simulink model "FAS_Kreuzungswarner_Simulation_V1"  (R2024b)
settings: Solver=FixedStepAuto  StartTime=0.0  StopTime=stoptime  FixedStep=sampletime  RelTol=1e-3
InitFcn:
  | if ~evalin('base', 'exist(''Auswertungsflag'', ''var'')') || evalin('base', 'Auswertungsflag.Value == 0')
  |     Parameterskript;
  |     run('StartGUI');  % explizit ausführen (nicht blockierend!)
  | end
values from neighbouring files (symbols this model uses):
  mEGO = str2double(massEGOInput.String)    [StartGUI.m]
  mFZG = str2double(massFZGInput.String)    [StartGUI.m]
  OeffnungswinkelA = str2double(angleInputA.String)    [StartGUI.m]
  OeffnungswinkelB = Simulink.Parameter    [Auswertung.m]    (also in StartGUI.m = str2double(angleInputB.String))
  P_EGO = str2double(powerEGOInput.String)    [StartGUI.m]
  P_FZG = str2double(powerFZGInput.String)    [StartGUI.m]
  ReichweiteA = str2double(rangeInputA.String)    [StartGUI.m]
  ReichweiteB = str2double(rangeInputB.String)    [StartGUI.m]
  SensorA = sensor1Dropdown.Value    [StartGUI.m]
  SensorB = sensor2Dropdown.Value    [StartGUI.m]
  startPositionEGO = str2double(posEGOInput.String)    [StartGUI.m]
  startPositionFzg = str2double(posFzgInput.String)    [StartGUI.m]
  v_EGO = str2double(velEGOInput.String)    [StartGUI.m]
  v_FZG = str2double(velFZGInput.String)    [StartGUI.m]
  Wetter = weatherDropdown.Value    [StartGUI.m]
  zweitesFzgSwitch = str2double(zweitesFzgInput.String)    [StartGUI.m]
undefined symbols (not defined in the file or in its folder): Airbagzeit, Ausloesezeit, b, dt, g, Haltezeit, l, munass, muschnee, mutrocken, rad_b, rad_l, reifen_dx, reifen_dy, SensorSwitch, startPositionFzg2, xFZG, yEGO
(part 2 of 3)

== matlab function FAS_Kreuzungswarner_Simulation_V1/FAF/MATLAB Function ==
  data: time input; Abstand input; GeschwindigkeitEGO input; Kollision input; Bremssignal input; Warnung input; defaultDistance parameter
%% Funktion zur Berechnung und Speicherung der für die Auswertung relevanten Parameter

% In dieser Funktion werden die für die Auswertung relevanten Parameter
% berechnet und danach im Workspace gespeichert sodass sie mit dem
% Auswertungsskript entsprechend gespeichert und dargestellt werden können

function Auswertung(time, Abstand, GeschwindigkeitEGO, Kollision, Bremssignal, Warnung, defaultDistance)
    
    persistent Kollisionszeitpunkt_gespeichert Erkennungszeitpunkt_gespeichert ReaktionszeitpunktWarnung_gespeichert ReaktionszeitpunktBremsung_gespeichert PufferzeitWarnung PufferzeitBremsung ...
                TimeToCollision Kollisionsgeschwindigkeit Kollisionszeitpunkt Erkennungszeitpunkt ReaktionszeitpunktWarnung ReaktionszeitpunktBremsung PufferAbstand

    % Variablen zur Berechnung der Zeitpunkte 
    if isempty(Kollisionszeitpunkt_gespeichert)
        Kollisionszeitpunkt_gespeichert = 0;
        Erkennungszeitpunkt_gespeichert = 0;
        ReaktionszeitpunktWarnung_gespeichert = 0;
        ReaktionszeitpunktBremsung_gespeichert = 0;
        Kollisionszeitpunkt = NaN;
        Erkennungszeitpunkt = NaN;
        ReaktionszeitpunktWarnung = NaN;
        ReaktionszeitpunktBremsung = NaN;
        PufferzeitWarnung = NaN;
        PufferzeitBremsung = NaN;
        TimeToCollision = NaN;
        Kollisionsgeschwindigkeit = NaN;
    end
    
    % Prüfung ob die Parameter einen Inhalt haben
    if isempty(PufferAbstand)
        PufferAbstand = defaultDistance;
    end

    if isempty(Kollisionszeitpunkt_gespeichert)
        Kollisionszeitpunkt_gespeichert = 0;
    end

    if isempty(Erkennungszeitpunkt_gespeichert)
        Erkennungszeitpunkt_gespeichert = 0;
    end

    if isempty(ReaktionszeitpunktWarnung_gespeichert)
        ReaktionszeitpunktWarnung_gespeichert = 0;
    end

    if isempty(ReaktionszeitpunktBremsung_gespeichert)
        ReaktionszeitpunktWarnung_gespeichert = 0;
    end
    
    % Wenn Kollision erkannt, Zeitpunkt nur einmal speichern
    if (Kollision > 0) && (Kollisionszeitpunkt_gespeichert == 0)
        Kollisionsgeschwindigkeit = GeschwindigkeitEGO * 3.6;
        Kollisionszeitpunkt = time;
        Kollisionszeitpunkt_gespeichert = 1;
    end

    % Erkennungszeitpunkt berechnen
    if (Abstand < defaultDistance) && (Erkennungszeitpunkt_gespeichert == 0)
        Erkennungszeitpunkt = time;
        Erkennungszeitpunkt_gespeichert = 1;
    end
    
    % Reaktionszeitpunkt für die Warnung berechnen
    if (Warnung > 0) && (ReaktionszeitpunktWarnung_gespeichert == 0)
        ReaktionszeitpunktWarnung = time;
        ReaktionszeitpunktWarnung_gespeichert = 1;
    end
    
    % Reaktionszeitpunkt für die Bremsung berechnen
    if (Bremssignal > 0) && (ReaktionszeitpunktBremsung_gespeichert == 0)
        ReaktionszeitpunktBremsung = time;
        ReaktionszeitpunktBremsung_gespeichert = 1;
    end    
    
    % Nur berechnen, wenn beide Zeitpunkte vorhanden sind
    if ~isnan(ReaktionszeitpunktWarnung) && ~isnan(Erkennungszeitpunkt)
        PufferzeitWarnung = ReaktionszeitpunktWarnung - Erkennungszeitpunkt;
    end

    if ~isnan(ReaktionszeitpunktBremsung) && ~isnan(Erkennungszeitpunkt)
        PufferzeitBremsung = ReaktionszeitpunktBremsung - Erkennungszeitpunkt;
    end
    
    if ~isnan(Kollisionszeitpunkt) && ~isnan(Erkennungszeitpunkt)
        TimeToCollision = Kollisionszeitpunkt - Erkennungszeitpunkt;
    end
    
    % Werte in Workspace schreiben (nur wenn diese gesetzt sind)
    if Kollisionszeitpunkt_gespeichert == 1
        assignin('base','Kollisionszeitpunkt',Kollisionszeitpunkt);
        assignin('base','Kollisionsgeschwindigkeit',Kollisionsgeschwindigkeit);
        Kollisionszeitpunkt_gespeichert = 2;
    end

    if Erkennungszeitpunkt_gespeichert == 1
        assignin('base','Erkennungszeitpunkt',Erkennungszeitpunkt);
        Erkennungszeitpunkt_gespeichert = 2;
    end

    if ReaktionszeitpunktWarnung_gespeichert == 1
        assignin('base','ReaktionszeitpunktWarnung',ReaktionszeitpunktWarnung);
        ReaktionszeitpunktWarnung_gespeichert = 2;
    end

    if ReaktionszeitpunktBremsung_gespeichert == 1
        assignin('base','ReaktionszeitpunktBremsung',ReaktionszeitpunktBremsung);
        ReaktionszeitpunktBremsung_gespeichert = 2;
    end

    if ~isnan(PufferzeitWarnung)
        assignin('base','PufferzeitWarnung',PufferzeitWarnung);
    end

    if ~isnan(PufferzeitBremsung)
        assignin('base','PufferzeitBremsung',PufferzeitBremsung);
    end
    
    % Werden auch bei NaN in den Workspace geschrieben da es Szenarien ohne
    % Crash gibt
    assignin('base','TimeToCollision',TimeToCollision);
    assignin('base','Kollisionszeitpunkt',Kollisionszeitpunkt);
    assignin('base','Kollisionsgeschwindigkeit',Kollisionsgeschwindigkeit);
    
    % PufferAbstand berechnen 
    if (PufferAbstand > Abstand)
        PufferAbstand = Abstand;
        assignin('base','PufferAbstand',PufferAbstand);
    end

== matlab function FAS_Kreuzungswarner_Simulation_V1/Sensor B/Radar/God Sensor mit Sichtfeld 1 ==
  data: xEGO input; yFzg input; distance output; collision output; yEGO parameter; xFZG parameter; b parameter; l parameter; OeffnungswinkelB parameter; ReichweiteB parameter
function [distance, collision] = abstand(xEGO, yFzg, yEGO, xFZG, b, l, OeffnungswinkelB, ReichweiteB)
    % Berechnung des Abstands zwischen EGO und Fzg, wenn Fzg sich im
    % Sichtfeld des EGO befindet

    % Initialisierung
    collision = 0;
    distance = 500;

    % Fahrzeugbegrenzungen berechnen
    x_min_Fzg = xFZG - b / 2;
    x_max_Fzg = xFZG + b / 2;
    y_min_Fzg = yFzg - l / 2;
    y_max_Fzg = yFzg + l / 2;
    x_min_EGO = xEGO - l / 2;
    x_max_EGO = xEGO + l / 2;
    y_min_EGO = yEGO - b / 2;
    y_max_EGO = yEGO + b / 2;

    % Kollisionsprüfung: Überlappung der Rechtecke?
    if (x_max_EGO >= x_min_Fzg && x_min_EGO <= x_max_Fzg) && ...
       (y_max_EGO >= y_min_Fzg && y_min_EGO <= y_max_Fzg)
        distance = 0;  
        collision = 10; % Kollision erkannt
        return
    end


    % Ecken + Kantenpunkte + Mittlepunkt des Fzg zur Sichtfeldprüfung
    testPoints = [
        linspace(x_min_Fzg, x_max_Fzg, 20)', repmat(y_min_Fzg, 20, 1); % Unterseite des Fzg
        linspace(x_min_Fzg, x_max_Fzg, 20)', repmat(y_max_Fzg, 20, 1); % Oberseite des Fzg
        repmat(x_min_Fzg, 18, 1), linspace(y_min_Fzg, y_max_Fzg, 18)'; % Linke Seite des Fzg
        repmat(x_max_Fzg, 18, 1), linspace(y_min_Fzg, y_max_Fzg, 18)'  % Rechte Seite des Fzg
        xFZG, yFzg % Mittelpunkt des Fzg
    ];

    % Sichtfeldprüfung: Mindestens ein Punkt im Sektor?
    isInside = false;
    for i = 1:size(testPoints,1)
        if isPointInSector(xEGO, yEGO, l, testPoints(i,1), testPoints(i,2), OeffnungswinkelB, ReichweiteB)
            isInside = true;
            break;
        end
    end

    if isInside
        if (collision ~= 10)
            % Messpunkte
            % EGO-Fahrzeug (horizontal ausgerichtet)
            top_EGO    = [linspace(x_min_EGO, x_max_EGO, 8)', repmat(y_max_EGO, 8, 1)];
            right_EGO  = [repmat(x_max_EGO, 8, 1), linspace(y_max_EGO, y_min_EGO, 8)'];
            bottom_EGO = [linspace(x_max_EGO, x_min_EGO, 8)', repmat(y_min_EGO, 8, 1)];
            left_EGO   = [repmat(x_min_EGO, 8, 1), linspace(y_min_EGO, y_max_EGO, 8)'];
            corners_EGO = [top_EGO; right_EGO; bottom_EGO; left_EGO];
    
            % Anderes Fahrzeug (vertikal ausgerichtet)
            top_Fzg    = [linspace(x_min_Fzg, x_max_Fzg, 8)', repmat(y_max_Fzg, 8, 1)];
            right_Fzg  = [repmat(x_max_Fzg, 8, 1), linspace(y_max_Fzg, y_min_Fzg, 8)'];
            bottom_Fzg = [linspace(x_max_Fzg, x_min_Fzg, 8)', repmat(y_min_Fzg, 8, 1)];
            left_Fzg   = [repmat(x_min_Fzg, 8, 1), linspace(y_min_Fzg, y_max_Fzg, 8)'];
            corners_Fzg = [top_Fzg; right_Fzg; bottom_Fzg; left_Fzg];
    
            % Abstand zwischen allen Punkten berechnen
            min_distance = inf;  
            for i = 1:32
                for j = 1:32
                    dx = corners_EGO(i,1) - corners_Fzg(j,1);
                    dy = corners_EGO(i,2) - corners_Fzg(j,2);
                    dist = sqrt(dx^2 + dy^2);
                    if dist < min_distance
                        min_distance = dist;
                    end
                end
            end
            distance = min_distance;
        end
    end
end

%% Sichtfeldprüfung für einen einzelnen Punkt
function isInside = isPointInSector(xEGO, yEGO, l, xP, yP, OeffnungswinkelB, ReichweiteB)
    % Prüft, ob der Punkt (xP, yP) im Sichtfeld des EGO liegt

    % Parameter
    OeffnungswinkelB = deg2rad(OeffnungswinkelB);
    alpha = -(OeffnungswinkelB/2);  % Startwinkel relativ zur x-Achse
    tol = max(1e-3, 1e-6 * ReichweiteB);

    % Mittelpunkt des Sektors
    xC = xEGO + l/2;
    yC = yEGO;

    % Richtungsvektor zum Punkt
    CP = [xP - xC, yP - yC];
    dist2 = CP(1)^2 + CP(2)^2;

    if dist2 > ReichweiteB^2 + tol
        isInside = false;
        return;
    end

    % Winkel vom Zentrum zum Punkt (in [-pi, pi])
    theta = atan2(CP(2), CP(1));  % atan2(y, x)

    % Endwinkel des Sichtfelds
    alphaEnd = alpha + OeffnungswinkelB;

    % Prüfung, ob Winkel theta im Sichtfeld liegt (inkl. Toleranz)
    isInside = (theta >= alpha - tol) && (theta <= alphaEnd + tol);
end

== matlab function FAS_Kreuzungswarner_Simulation_V1/Fahrdynamik/MATLAB Function ==
  data: VorgabeGeschwindigkeitEGO input; Anfahrgeschwindigkeit input; GeschwindigkeitEGO input; Geschwindigkeit_EGOneudelay input; Geschwindigkeit_EGOneu output
%% Berechnung der Geschwindigkeit des EGOs beim Anfahren

% Es wird die aktuelle Geschwindigkeit gespeichert solang sie niedriger ist
% als die Gschwindigkeit aus dem vorigen Simulationsschritt. Die minimale
% Geschwindigkeit wird gespeichert und mit der aktuellen
% Anfahrgeschwindigkeit verrechnet

function Geschwindigkeit_EGOneu = Geschwindigkeitsberechnung(VorgabeGeschwindigkeitEGO, Anfahrgeschwindigkeit, GeschwindigkeitEGO, Geschwindigkeit_EGOneudelay)

persistent Counter DummyGeschwindigkeit

% Prüfung ob Parameter schon einen Inhalt haben
if isempty(Counter)
    Counter = 0;
end

if isempty(DummyGeschwindigkeit)
    DummyGeschwindigkeit = 100000000;
end

% Prüfung ob die aktuelle Geschwindigkeit kleiner als die davor ist
if (DummyGeschwindigkeit > GeschwindigkeitEGO)
    DummyGeschwindigkeit = GeschwindigkeitEGO;
end

% Counter erhöhen, da der Integrator vor dem Berechnen nochmal auf 0
% gesetzt wird
if(Anfahrgeschwindigkeit == 0)
    Counter = Counter + 1;
end

% Verrechnen mit der Anfahrgeschwindigkeit beim Anfahren nach dem
% Bremsvorgang
if(Counter > 1 && VorgabeGeschwindigkeitEGO > Geschwindigkeit_EGOneudelay)
    Geschwindigkeit_EGOneu = Anfahrgeschwindigkeit + DummyGeschwindigkeit;
else
    Geschwindigkeit_EGOneu = GeschwindigkeitEGO;
end

== matlab function FAS_Kreuzungswarner_Simulation_V1/Sensor A/C2X/God Sensor mit Sichtfeld ==
  data: xEGO input; yFzg input; distance output; collision output; yEGO parameter; xFZG parameter; b parameter; l parameter; ReichweiteA parameter; relevanz input; OeffnungswinkelA parameter
function [distance, collision] = abstand(xEGO, yFzg, yEGO, xFZG, b, l, ReichweiteA, relevanz, OeffnungswinkelA)
    % Berechnung des Abstands zwischen EGO und Fzg, wenn Fzg sich im
    % Sichtfeld des EGO befindet
    % Initialisierung
    collision = 0;
    distance = 500;
    
    if relevanz == 1
        % Fahrzeugbegrenzungen berechnen
        x_min_Fzg = xFZG - b / 2;
        x_max_Fzg = xFZG + b / 2;
        y_min_Fzg = yFzg - l / 2;
        y_max_Fzg = yFzg + l / 2;
        x_min_EGO = xEGO - l / 2;
        x_max_EGO = xEGO + l / 2;
        y_min_EGO = yEGO - b / 2;
        y_max_EGO = yEGO + b / 2;

        % Kollisionsprüfung: Überlappung der Rechtecke?
        if (x_max_EGO >= x_min_Fzg && x_min_EGO <= x_max_Fzg) && ...
           (y_max_EGO >= y_min_Fzg && y_min_EGO <= y_max_Fzg)
            distance = 0;  
            collision = 10; % Kollision erkannt
            return
        end
    
        % Ecken + Kantenpunkte + Mittlepunkt des Fzg zur Sichtfeldprüfung
        testPoints = [
            linspace(x_min_Fzg, x_max_Fzg, 20)', repmat(y_min_Fzg, 20, 1); % Unterseite des Fzg
            linspace(x_min_Fzg, x_max_Fzg, 20)', repmat(y_max_Fzg, 20, 1); % Oberseite des Fzg
            repmat(x_min_Fzg, 18, 1), linspace(y_min_Fzg, y_max_Fzg, 18)'; % Linke Seite des Fzg
            repmat(x_max_Fzg, 18, 1), linspace(y_min_Fzg, y_max_Fzg, 18)'  % Rechte Seite des Fzg
            xFZG, yFzg % Mittelpunkt des Fzg
        ];
    
        % Sichtfeldprüfung: Mindestens ein Punkt im Sektor?
        isInside = false;
        for i = 1:size(testPoints,1)
            if isPointInSector(xEGO, yEGO, l, testPoints(i,1), testPoints(i,2), OeffnungswinkelA, ReichweiteA)
                isInside = true;
                break;
            end
        end
    
        if isInside
            if(collision ~= 10)
                % Messpunkte
                % EGO-Fahrzeug (horizontal ausgerichtet)
                top_EGO    = [linspace(x_min_EGO, x_max_EGO, 8)', repmat(y_max_EGO, 8, 1)];
                right_EGO  = [repmat(x_max_EGO, 8, 1), linspace(y_max_EGO, y_min_EGO, 8)'];
                bottom_EGO = [linspace(x_max_EGO, x_min_EGO, 8)', repmat(y_min_EGO, 8, 1)];
                left_EGO   = [repmat(x_min_EGO, 8, 1), linspace(y_min_EGO, y_max_EGO, 8)'];
                corners_EGO = [top_EGO; right_EGO; bottom_EGO; left_EGO];
        
                % Anderes Fahrzeug (vertikal ausgerichtet)
                top_Fzg    = [linspace(x_min_Fzg, x_max_Fzg, 8)', repmat(y_max_Fzg, 8, 1)];
                right_Fzg  = [repmat(x_max_Fzg, 8, 1), linspace(y_max_Fzg, y_min_Fzg, 8)'];
                bottom_Fzg = [linspace(x_max_Fzg, x_min_Fzg, 8)', repmat(y_min_Fzg, 8, 1)];
                left_Fzg   = [repmat(x_min_Fzg, 8, 1), linspace(y_min_Fzg, y_max_Fzg, 8)'];
                corners_Fzg = [top_Fzg; right_Fzg; bottom_Fzg; left_Fzg];
        
                % Abstand zwischen allen Punkten berechnen
                min_distance = inf;  
                for i = 1:32
                    for j = 1:32
                        dx = corners_EGO(i,1) - corners_Fzg(j,1);
                        dy = corners_EGO(i,2) - corners_Fzg(j,2);
                        dist = sqrt(dx^2 + dy^2);
                        if dist < min_distance
                            min_distance = dist;
                        end
                    end
                end
                distance = min_distance;
            end
        end
    end
end

%% Sichtfeldprüfung für einen einzelnen Punkt
function isInside = isPointInSector(xEGO, yEGO, l, xP, yP, OeffnungswinkelA, ReichweiteA)
    % Prüft, ob der Punkt (xP, yP) im Sichtfeld des EGO liegt

    % Parameter
    OeffnungswinkelA = deg2rad(OeffnungswinkelA);
    alpha = -(OeffnungswinkelA/2);  % Startwinkel relativ zur x-Achse
    tol = max(1e-3, 1e-6 * ReichweiteA);

    % Mittelpunkt des Sektors
    xC = xEGO + l/2;
    yC = yEGO;

    % Richtungsvektor zum Punkt
    CP = [xP - xC, yP - yC];
    dist2 = CP(1)^2 + CP(2)^2;

    if dist2 > ReichweiteA^2 + tol
        isInside = false;
        return;
    end

    % Winkel vom Zentrum zum Punkt (in [-pi, pi])
    theta = atan2(CP(2), CP(1));  % atan2(y, x)

    % Endwinkel des Sichtfelds
    alphaEnd = alpha + OeffnungswinkelA;

    % Prüfung, ob Winkel theta im Sichtfeld liegt (inkl. Toleranz)
    isInside = (theta >= alpha - tol) && (theta <= alphaEnd + tol);
end

== matlab function FAS_Kreuzungswarner_Simulation_V1/Sensor A/C2X/Relevanz Kontrolle/Bewegungs-Achse Fzg ==
  data: xFzg input; bewegung output; xFzg_prev input; yFzg input; yFzg_prev input
function bewegung = fcn(xFzg, xFzg_prev, yFzg, yFzg_prev)
% Prüfung ob Fzg eine Bewegung in X oder Y Richtung hat 
% X Bewegung: bewegung = 1
% Y Bewegung: bewegung = 2
% X&Y Bewegung: bewegung = 3
% Keine Bewegung: bewegung = 0

    if xFzg ~= xFzg_prev
        xBewegung = 1;
    else
        xBewegung = 0;
    end

    if yFzg  ~= yFzg_prev
        yBewegung = 2;
    else
        yBewegung = 0;
    end

    bewegung = xBewegung + yBewegung;

end

== matlab function FAS_Kreuzungswarner_Simulation_V1/Sensor A/C2X/Relevanz Kontrolle/Logik ==
  data: outY input; distance input; outX input; relevanz output; defaultDistance parameter
function relevanz = direction(outY, distance, outX, defaultDistance)
% Wenn der Sensor ein fzg erkennt (distance < defaultDistance) Wir wenn
% EGO und Fzg noch vor der Kreuzung sind eine Relevanz ausgegeben (1). Wenn
% nicht wird das Fzg als nicht Relevant gemarkt (-1)

    if distance < defaultDistance 
        if outX == 1 && outY == 1
            relevanz = 1;
        else
            relevanz = -1;
        end
    else
        relevanz = 0;
    end

end

== matlab function FAS_Kreuzungswarner_Simulation_V1/Sensor A/C2X/Relevanz Kontrolle/Relevanz Kreuzung x ==
  data: xPos input; out output; xPos_prev input; targetX input; b parameter
function out = direction(xPos, xPos_prev, targetX, b)
% Gibt 1 aus, wenn sich das Rechteck zubewegt oder innerhalb 4.25 ist
% Gibt -1 aus, wenn es sich entfernt und weiter als 4.25 ist
% Gibt 0 aus, wenn es genau auf dem Punkt ist

    % Berechne die Distanz des Rechtecks zum Zielpunkt targetY
    dist = abs(xPos - targetX);
    dist_prev = abs(xPos_prev - targetX);

    % Bewegungsrichtung des Rechtecks
    delta = dist - dist_prev;

    % Überprüfe die Bedingungen basierend auf der Bewegungsrichtung
    if dist <= b
        out = 1; % Rechteck bewegt sich auf den Punkt zu oder ist nah genug dran
    elseif delta < 0
        out = 1; % Rechteck bewegt sich auf den Punkt zu
    else
        out = -1; % Rechteck entfernt sich vom Punkt
    end
end

== matlab function FAS_Kreuzungswarner_Simulation_V1/Sensor A/C2X/Relevanz Kontrolle/Relevanz Kreuzung y ==
  data: yPos input; out output; yPos_prev input; targetY input; b parameter
function out = direction(yPos, yPos_prev, targetY, b)
% Gibt 1 aus, wenn sich das Rechteck zubewegt oder innerhalb 4.25 ist
% Gibt -1 aus, wenn es sich entfernt und weiter als 4.25 ist
% Gibt 0 aus, wenn es genau auf dem Punkt ist

    % Berechne die Distanz des Rechtecks zum Zielpunkt targetY
    dist = abs(yPos - targetY);
    dist_prev = abs(yPos_prev - targetY);

    % Bewegungsrichtung des Rechtecks
    delta = dist - dist_prev;

    % Überprüfe die Bedingungen basierend auf der Bewegungsrichtung
    if dist <= b
        out = 1; % Rechteck bewegt sich auf den Punkt zu oder ist nah genug dran
    elseif delta < 0
        out = 1; % Rechteck bewegt sich auf den Punkt zu
    else
        out = -1; % Rechteck entfernt sich vom Punkt
    end
end

== matlab function FAS_Kreuzungswarner_Simulation_V1/Sensor A/God Sensor/God Sensor ==
  data: xEGO input; yFzg input; distance output; collision output; yEGO parameter; xFZG parameter; b parameter; l parameter
function [distance, collision] = fcn(xEGO, yFzg, yEGO, xFZG, b, l)

    collision = 0;

    % Fahrzeugbegrenzungen berechnen
    x_min_EGO = xEGO - l / 2;
    x_max_EGO = xEGO + l / 2;
    y_min_EGO = yEGO - b / 2;
    y_max_EGO = yEGO + b / 2;

    x_min_Fzg = xFZG - b / 2;
    x_max_Fzg = xFZG + b / 2;
    y_min_Fzg = yFzg - l / 2;
    y_max_Fzg = yFzg + l / 2;

    % Kollisionsprüfung: Überlappen sich die Rechtecke?
    if (x_max_EGO >= x_min_Fzg && x_min_EGO <= x_max_Fzg) && ...
       (y_max_EGO >= y_min_Fzg && y_min_EGO <= y_max_Fzg)
        distance = 0;  
        collision = 10; % Kollision erkannt
        return
    else
        % Messpunkte
        % EGO-Fahrzeug (horizontal ausgerichtet)
        top_EGO    = [linspace(x_min_EGO, x_max_EGO, 8)', repmat(y_max_EGO, 8, 1)];
        right_EGO  = [repmat(x_max_EGO, 8, 1), linspace(y_max_EGO, y_min_EGO, 8)'];
        bottom_EGO = [linspace(x_max_EGO, x_min_EGO, 8)', repmat(y_min_EGO, 8, 1)];
        left_EGO   = [repmat(x_min_EGO, 8, 1), linspace(y_min_EGO, y_max_EGO, 8)'];
        corners_EGO = [top_EGO; right_EGO; bottom_EGO; left_EGO];

        % Anderes Fahrzeug (vertikal ausgerichtet)
        top_Fzg    = [linspace(x_min_Fzg, x_max_Fzg, 8)', repmat(y_max_Fzg, 8, 1)];
        right_Fzg  = [repmat(x_max_Fzg, 8, 1), linspace(y_max_Fzg, y_min_Fzg, 8)'];
        bottom_Fzg = [linspace(x_max_Fzg, x_min_Fzg, 8)', repmat(y_min_Fzg, 8, 1)];
        left_Fzg   = [repmat(x_min_Fzg, 8, 1), linspace(y_min_Fzg, y_max_Fzg, 8)'];
        corners_Fzg = [top_Fzg; right_Fzg; bottom_Fzg; left_Fzg];

        % Abstand zwischen allen Punkten berechnen
        min_distance = inf;  
        for i = 1:32
            for j = 1:32
                dx = corners_EGO(i,1) - corners_Fzg(j,1);
                dy = corners_EGO(i,2) - corners_Fzg(j,2);
                dist = sqrt(dx^2 + dy^2);
                if dist < min_distance
                    min_distance = dist;
                end
            end
        end
        distance = min_distance;
    end
end

== matlab function FAS_Kreuzungswarner_Simulation_V1/Sensor A/God Sensor/Relevanz Kontrolle/Bewegungs-Achse Fzg ==
  data: xFzg input; bewegung output; xFzg_prev input; yFzg input; yFzg_prev input
function bewegung = fcn(xFzg, xFzg_prev, yFzg, yFzg_prev)
% Prüfung ob Fzg eine Bewegung in X oder Y Richtung hat 
% X Bewegung: bewegung = 1
% Y Bewegung: bewegung = 2
% X&Y Bewegung: bewegung = 3
% Keine Bewegung: bewegung = 0

    if xFzg ~= xFzg_prev
        xBewegung = 1;
    else
        xBewegung = 0;
    end

    if yFzg  ~= yFzg_prev
        yBewegung = 2;
    else
        yBewegung = 0;
    end

    bewegung = xBewegung + yBewegung;

end

== matlab function FAS_Kreuzungswarner_Simulation_V1/Fahrdynamik/MATLAB Function1 ==
  data: Anfahrbeschleunigung output; mutrocken parameter; munass parameter; mEGO parameter; P_EGO parameter; g parameter; Geschwindigkeit_EGOneu input; Wetter parameter; muschnee parameter
%% Berechnung eines realistischen Anfahrens nach dem Bremsvorgang

% In Abhängigkeit vom aktuellen Reibwert der Straße, dem Schlupf, dem 
% Wirkungsgrad und dem maximalen Motormoment werden zwei mögliche 
% Beschleunigungen errechnet. Es wird immer die niedrigere Beschleunigung
% genommen da entweder das eine physikalisch nicht möglich oder das andere
% vom Motor aktuell nicht lieferbar ist. 

function Anfahrbeschleunigung = MaxBeschleunigung(mutrocken, munass, mEGO, P_EGO, g, Geschwindigkeit_EGOneu, Wetter, muschnee)

    % Reibwert bestimmen
    mu = mutrocken;
    if Wetter == 2
        mu = munass * (0.7 + 0.3 * min(Geschwindigkeit_EGOneu / 10, 1));
    elseif Wetter == 3
        mu = muschnee * (0.7 + 0.3 * min(Geschwindigkeit_EGOneu / 10, 1));
    end

    % Effektiver Reibwert mit schlupfbedingter Reduktion bei niedrigen Geschwindigkeiten
    if Wetter == 2 || Wetter == 3
        schlupfFaktor = 0.5 + 0.5 * min(Geschwindigkeit_EGOneu / 5, 1);  % zwischen 0.5 (Stillstand) und 1.0
    else
        schlupfFaktor = 0.7 + 0.3 * min(Geschwindigkeit_EGOneu / 5, 1);  % weniger Reduktion bei Trockenheit
    end
    
    mu_effektiv = mu * schlupfFaktor;


    % Geschwindigkeitsabhängiger Wirkungsgrad
    if (Geschwindigkeit_EGOneu <= 5)
        eta = 0.3;
    elseif (Geschwindigkeit_EGOneu <= 10)
        eta = 0.5;
    else
        eta = 0.8;
    end
    
    % Berechnung verschiedene Beschleunigung Begrenzung auf realistisch
    % maximale 3.5 m/s^2 um es sanft / angenehm zu haben
    begrenzteBeschleunigung = 3.5;
    maxBeschleunigung = mu_effektiv * g;

    if (Geschwindigkeit_EGOneu < 1.0)
          Geschwindigkeit_EGOneu = 1.0;
    end

    Motorbeschleunigung = (P_EGO * 1000 * eta) / (mEGO * Geschwindigkeit_EGOneu);
    
    % Prüfung ob Beschleunigung überhaupt möglich ist mit dem aktuellen mu
    realistisch = min(maxBeschleunigung, Motorbeschleunigung);
    Anfahrbeschleunigung = min(begrenzteBeschleunigung, realistisch);
end

== matlab function FAS_Kreuzungswarner_Simulation_V1/Sensor A/God Sensor/Relevanz Kontrolle/Relevanz Kreuzung x ==
  data: xPos input; out output; xPos_prev input; targetX input; b parameter
function out = direction(xPos, xPos_prev, targetX, b)
% Gibt 1 aus, wenn sich das Rechteck zubewegt oder innerhalb 4.25 ist
% Gibt -1 aus, wenn es sich entfernt und weiter als 4.25 ist
% Gibt 0 aus, wenn es genau auf dem Punkt ist

    % Berechne die Distanz des Rechtecks zum Zielpunkt targetY
    dist = abs(xPos - targetX);
    dist_prev = abs(xPos_prev - targetX);

    % Bewegungsrichtung des Rechtecks
    delta = dist - dist_prev;

    % Überprüfe die Bedingungen basierend auf der Bewegungsrichtung
    if dist <= b
        out = 1; % Rechteck bewegt sich auf den Punkt zu oder ist nah genug dran
    elseif delta < 0
        out = 1; % Rechteck bewegt sich auf den Punkt zu
    else
        out = -1; % Rechteck entfernt sich vom Punkt
    end
end

== matlab function FAS_Kreuzungswarner_Simulation_V1/Sensor A/God Sensor/Relevanz Kontrolle/Relevanz Kreuzung y ==
  data: yPos input; out output; yPos_prev input; targetY input; b parameter
function out = direction(yPos, yPos_prev, targetY, b)
% Gibt 1 aus, wenn sich das Rechteck zubewegt oder innerhalb 4.25 ist
% Gibt -1 aus, wenn es sich entfernt und weiter als 4.25 ist
% Gibt 0 aus, wenn es genau auf dem Punkt ist

    % Berechne die Distanz des Rechtecks zum Zielpunkt targetY
    dist = abs(yPos - targetY);
    dist_prev = abs(yPos_prev - targetY);

    % Bewegungsrichtung des Rechtecks
    delta = dist - dist_prev;

    % Überprüfe die Bedingungen basierend auf der Bewegungsrichtung
    if dist <= b
        out = 1; % Rechteck bewegt sich auf den Punkt zu oder ist nah genug dran
    elseif delta < 0
        out = 1; % Rechteck bewegt sich auf den Punkt zu
    else
        out = -1; % Rechteck entfernt sich vom Punkt
    end
end

== matlab function FAS_Kreuzungswarner_Simulation_V1/Sensor A/Relevanz Kontrolle/Bewegungs-Achse Fzg1 ==
  data: xFzg input; bewegung output; xFzg_prev input; yFzg input; yFzg_prev input
function bewegung = fcn(xFzg, xFzg_prev, yFzg, yFzg_prev)
% Prüfung ob Fzg eine Bewegung in X oder Y Richtung hat 
% X Bewegung: bewegung = 1
% Y Bewegung: bewegung = 2
% X&Y Bewegung: bewegung = 3
% Keine Bewegung: bewegung = 0

    if xFzg ~= xFzg_prev
        xBewegung = 1;
    else
        xBewegung = 0;
    end

    if yFzg  ~= yFzg_prev
        yBewegung = 2;
    else
        yBewegung = 0;
    end

    bewegung = xBewegung + yBewegung;

end

== matlab function FAS_Kreuzungswarner_Simulation_V1/Sensor A/Sensor Switch ==
  data: selection input; distance output; distanceG input; collisionG input; relevanzG input; distanceC2X input; collisionC2X input; collision output; relevanzC2X input; relevanz output
function [distance, collision, relevanz] = sensorSwitch(selection, ...
                                                        distanceG, collisionG, relevanzG, ...
                                                        distanceC2X, collisionC2X, relevanzC2X)
   

    switch selection
        case 1
            distance = distanceC2X;
            collision = collisionC2X;
            relevanz = relevanzC2X;
        
        case 2
            distance = distanceG;
            collision = collisionG;
            relevanz = relevanzG;


        % Wenn kein Sensor ausgewält ist
        case 3
            distance = 500;
            collision = 0;
            relevanz = 0;         
            
        otherwise
            distance = -100; %Fehler
            collision = -100; %Fehler
            relevanz = -100; %Fehler
    end
end

== matlab function FAS_Kreuzungswarner_Simulation_V1/Sensor B/Kamera/God Sensor mit Sichtfeld  ==
  data: xEGO input; yFzg input; distance output; collision output; yEGO parameter; xFZG parameter; b parameter; l parameter; OeffnungswinkelB parameter; ReichweiteB parameter
function [distance, collision] = abstand(xEGO, yFzg, yEGO, xFZG, b, l, OeffnungswinkelB, ReichweiteB)
    % Berechnung des Abstands zwischen EGO und Fzg, wenn Fzg sich im
    % Sichtfeld des EGO befindet

    % Initialisierung
    collision = 0;
    distance = 500;

    % Fahrzeugbegrenzungen berechnen
    x_min_Fzg = xFZG - b / 2;
    x_max_Fzg = xFZG + b / 2;
    y_min_Fzg = yFzg - l / 2;
    y_max_Fzg = yFzg + l / 2;
    x_min_EGO = xEGO - l / 2;
    x_max_EGO = xEGO + l / 2;
    y_min_EGO = yEGO - b / 2;
    y_max_EGO = yEGO + b / 2;

    % Kollisionsprüfung: Überlappung der Rechtecke?
    if (x_max_EGO >= x_min_Fzg && x_min_EGO <= x_max_Fzg) && ...
       (y_max_EGO >= y_min_Fzg && y_min_EGO <= y_max_Fzg)
        distance = 0;  
        collision = 10; % Kollision erkannt
        return
    end


    % Ecken + Kantenpunkte + Mittlepunkt des Fzg zur Sichtfeldprüfung
    testPoints = [
        linspace(x_min_Fzg, x_max_Fzg, 20)', repmat(y_min_Fzg, 20, 1); % Unterseite des Fzg
        linspace(x_min_Fzg, x_max_Fzg, 20)', repmat(y_max_Fzg, 20, 1); % Oberseite des Fzg
        repmat(x_min_Fzg, 18, 1), linspace(y_min_Fzg, y_max_Fzg, 18)'; % Linke Seite des Fzg
        repmat(x_max_Fzg, 18, 1), linspace(y_min_Fzg, y_max_Fzg, 18)'  % Rechte Seite des Fzg
        xFZG, yFzg % Mittelpunkt des Fzg
    ];

    % Sichtfeldprüfung: Mindestens ein Punkt im Sektor?
    isInside = false;
    for i = 1:size(testPoints,1)
        if isPointInSector(xEGO, yEGO, l, testPoints(i,1), testPoints(i,2), OeffnungswinkelB, ReichweiteB)
            isInside = true;
            break;
        end
    end

    if isInside
        if (collision ~= 10)
            % Messpunkte
            % EGO-Fahrzeug (horizontal ausgerichtet)
            top_EGO    = [linspace(x_min_EGO, x_max_EGO, 8)', repmat(y_max_EGO, 8, 1)];
            right_EGO  = [repmat(x_max_EGO, 8, 1), linspace(y_max_EGO, y_min_EGO, 8)'];
            bottom_EGO = [linspace(x_max_EGO, x_min_EGO, 8)', repmat(y_min_EGO, 8, 1)];
            left_EGO   = [repmat(x_min_EGO, 8, 1), linspace(y_min_EGO, y_max_EGO, 8)'];
            corners_EGO = [top_EGO; right_EGO; bottom_EGO; left_EGO];
    
            % Anderes Fahrzeug (vertikal ausgerichtet)
            top_Fzg    = [linspace(x_min_Fzg, x_max_Fzg, 8)', repmat(y_max_Fzg, 8, 1)];
            right_Fzg  = [repmat(x_max_Fzg, 8, 1), linspace(y_max_Fzg, y_min_Fzg, 8)'];
            bottom_Fzg = [linspace(x_max_Fzg, x_min_Fzg, 8)', repmat(y_min_Fzg, 8, 1)];
            left_Fzg   = [repmat(x_min_Fzg, 8, 1), linspace(y_min_Fzg, y_max_Fzg, 8)'];
            corners_Fzg = [top_Fzg; right_Fzg; bottom_Fzg; left_Fzg];
    
            % Abstand zwischen allen Punkten berechnen
            min_distance = inf;  
            for i = 1:32
                for j = 1:32
                    dx = corners_EGO(i,1) - corners_Fzg(j,1);
                    dy = corners_EGO(i,2) - corners_Fzg(j,2);
                    dist = sqrt(dx^2 + dy^2);
                    if dist < min_distance
                        min_distance = dist;
                    end
                end
            end
            distance = min_distance;
        end
    end
end

%% Sichtfeldprüfung für einen einzelnen Punkt
function isInside = isPointInSector(xEGO, yEGO, l, xP, yP, OeffnungswinkelB, ReichweiteB)
    % Prüft, ob der Punkt (xP, yP) im Sichtfeld des EGO liegt

    % Parameter
    OeffnungswinkelB = deg2rad(OeffnungswinkelB);
    alpha = -(OeffnungswinkelB/2);  % Startwinkel relativ zur x-Achse
    tol = max(1e-3, 1e-6 * ReichweiteB);

    % Mittelpunkt des Sektors
    xC = xEGO + l/2;
    yC = yEGO;

    % Richtungsvektor zum Punkt
    CP = [xP - xC, yP - yC];
    dist2 = CP(1)^2 + CP(2)^2;

    if dist2 > ReichweiteB^2 + tol
        isInside = false;
        return;
    end

    % Winkel vom Zentrum zum Punkt (in [-pi, pi])
    theta = atan2(CP(2), CP(1));  % atan2(y, x)

    % Endwinkel des Sichtfelds
    alphaEnd = alpha + OeffnungswinkelB;

    % Prüfung, ob Winkel theta im Sichtfeld liegt (inkl. Toleranz)
    isInside = (theta >= alpha - tol) && (theta <= alphaEnd + tol);
end

== matlab function FAS_Kreuzungswarner_Simulation_V1/Sensor B/Kamera/Relevanz Kontrolle/Bewegungs-Achse Fzg ==
  data: xFzg input; bewegung output; xFzg_prev input; yFzg input; yFzg_prev input
function bewegung = fcn(xFzg, xFzg_prev, yFzg, yFzg_prev)
% Prüfung ob Fzg eine Bewegung in X oder Y Richtung hat 
% X Bewegung: bewegung = 1
% Y Bewegung: bewegung = 2
% X&Y Bewegung: bewegung = 3
% Keine Bewegung: bewegung = 0

    if xFzg ~= xFzg_prev
        xBewegung = 1;
    else
        xBewegung = 0;
    end

    if yFzg  ~= yFzg_prev
        yBewegung = 2;
    else
        yBewegung = 0;
    end

    bewegung = xBewegung + yBewegung;

end

== matlab function FAS_Kreuzungswarner_Simulation_V1/Sensor B/Kamera/Relevanz Kontrolle/Logik ==
  data: outY input; distance input; outX input; relevanz output; defaultDistance parameter
function relevanz = direction(outY, distance, outX, defaultDistance)
% Wenn der Sensor ein fzg erkennt (distance < defaultDistance) Wir wenn
% EGO und Fzg noch vor der Kreuzung sind eine Relevanz ausgegeben (1). Wenn
% nicht wird das Fzg als nicht Relevant gemarkt (-1)

    if distance < defaultDistance 
        if outX == 1 && outY == 1
            relevanz = 1;
        else
            relevanz = -1;
        end
    else
        relevanz = 0;
    end

end

== matlab function FAS_Kreuzungswarner_Simulation_V1/Sensor B/Kamera/Relevanz Kontrolle/Relevanz Kreuzung x ==
  data: xPos input; out output; xPos_prev input; targetX input; b parameter
function out = direction(xPos, xPos_prev, targetX, b)
% Gibt 1 aus, wenn sich das Rechteck zubewegt oder innerhalb 4.25 ist
% Gibt -1 aus, wenn es sich entfernt und weiter als 4.25 ist
% Gibt 0 aus, wenn es genau auf dem Punkt ist

    % Berechne die Distanz des Rechtecks zum Zielpunkt targetY
    dist = abs(xPos - targetX);
    dist_prev = abs(xPos_prev - targetX);

    % Bewegungsrichtung des Rechtecks
    delta = dist - dist_prev;

    % Überprüfe die Bedingungen basierend auf der Bewegungsrichtung
    if dist <= b
        out = 1; % Rechteck bewegt sich auf den Punkt zu oder ist nah genug dran
    elseif delta < 0
        out = 1; % Rechteck bewegt sich auf den Punkt zu
    else
        out = -1; % Rechteck entfernt sich vom Punkt
    end
end

== matlab function FAS_Kreuzungswarner_Simulation_V1/Sensor B/Kamera/Relevanz Kontrolle/Relevanz Kreuzung y ==
  data: yPos input; out output; yPos_prev input; targetY input; b parameter
function out = direction(yPos, yPos_prev, targetY, b)
% Gibt 1 aus, wenn sich das Rechteck zubewegt oder innerhalb 4.25 ist
% Gibt -1 aus, wenn es sich entfernt und weiter als 4.25 ist
% Gibt 0 aus, wenn es genau auf dem Punkt ist

    % Berechne die Distanz des Rechtecks zum Zielpunkt targetY
    dist = abs(yPos - targetY);
    dist_prev = abs(yPos_prev - targetY);

    % Bewegungsrichtung des Rechtecks
    delta = dist - dist_prev;

    % Überprüfe die Bedingungen basierend auf der Bewegungsrichtung
    if dist <= b
        out = 1; % Rechteck bewegt sich auf den Punkt zu oder ist nah genug dran
    elseif delta < 0
        out = 1; % Rechteck bewegt sich auf den Punkt zu
    else
        out = -1; % Rechteck entfernt sich vom Punkt
    end
end

== matlab function FAS_Kreuzungswarner_Simulation_V1/Sensor B/Radar/Relevanz Kontrolle/Bewegungs-Achse Fzg ==
  data: xFzg input; bewegung output; xFzg_prev input; yFzg input; yFzg_prev input
function bewegung = fcn(xFzg, xFzg_prev, yFzg, yFzg_prev)
% Prüfung ob Fzg eine Bewegung in X oder Y Richtung hat 
% X Bewegung: bewegung = 1
% Y Bewegung: bewegung = 2
% X&Y Bewegung: bewegung = 3
% Keine Bewegung: bewegung = 0

    if xFzg ~= xFzg_prev
        xBewegung = 1;
    else
        xBewegung = 0;
    end

    if yFzg  ~= yFzg_prev
        yBewegung = 2;
    else
        yBewegung = 0;
    end

    bewegung = xBewegung + yBewegung;

end

== matlab function FAS_Kreuzungswarner_Simulation_V1/Sensor B/Radar/Relevanz Kontrolle/Logik ==
  data: outY input; distance input; outX input; relevanz output; defaultDistance parameter
function relevanz = direction(outY, distance, outX, defaultDistance)
% Wenn der Sensor ein fzg erkennt (distance < defaultDistance) Wir wenn
% EGO und Fzg noch vor der Kreuzung sind eine Relevanz ausgegeben (1). Wenn
% nicht wird das Fzg als nicht Relevant gemarkt (-1)

    if distance < defaultDistance 
        if outX == 1 && outY == 1
            relevanz = 1;
        else
            relevanz = -1;
        end
    else
        relevanz = 0;
    end

end

== matlab function FAS_Kreuzungswarner_Simulation_V1/Sensor B/Radar/Relevanz Kontrolle/Relevanz Kreuzung x ==
  data: xPos input; out output; xPos_prev input; targetX input; b parameter
function out = direction(xPos, xPos_prev, targetX, b)
% Gibt 1 aus, wenn sich das Rechteck zubewegt oder innerhalb 4.25 ist
% Gibt -1 aus, wenn es sich entfernt und weiter als 4.25 ist
% Gibt 0 aus, wenn es genau auf dem Punkt ist

    % Berechne die Distanz des Rechtecks zum Zielpunkt targetY
    dist = abs(xPos - targetX);
    dist_prev = abs(xPos_prev - targetX);

    % Bewegungsrichtung des Rechtecks
    delta = dist - dist_prev;

    % Überprüfe die Bedingungen basierend auf der Bewegungsrichtung
    if dist <= b
        out = 1; % Rechteck bewegt sich auf den Punkt zu oder ist nah genug dran
    elseif delta < 0
        out = 1; % Rechteck bewegt sich auf den Punkt zu
    else
        out = -1; % Rechteck entfernt sich vom Punkt
    end
end

== matlab function FAS_Kreuzungswarner_Simulation_V1/Sensor B/Radar/Relevanz Kontrolle/Relevanz Kreuzung y ==
  data: yPos input; out output; yPos_prev input; targetY input; b parameter
function out = direction(yPos, yPos_prev, targetY, b)
% Gibt 1 aus, wenn sich das Rechteck zubewegt oder innerhalb 4.25 ist
% Gibt -1 aus, wenn es sich entfernt und weiter als 4.25 ist
% Gibt 0 aus, wenn es genau auf dem Punkt ist

    % Berechne die Distanz des Rechtecks zum Zielpunkt targetY
    dist = abs(yPos - targetY);
    dist_prev = abs(yPos_prev - targetY);

    % Bewegungsrichtung des Rechtecks
    delta = dist - dist_prev;

    % Überprüfe die Bedingungen basierend auf der Bewegungsrichtung
    if dist <= b
        out = 1; % Rechteck bewegt sich auf den Punkt zu oder ist nah genug dran
    elseif delta < 0
        out = 1; % Rechteck bewegt sich auf den Punkt zu
    else
        out = -1; % Rechteck entfernt sich vom Punkt
    end
end

== matlab function FAS_Kreuzungswarner_Simulation_V1/Sensor B/Relevanz Kontrolle/Bewegungs-Achse Fzg1 ==
  data: xFzg input; bewegung output; xFzg_prev input; yFzg input; yFzg_prev input
function bewegung = fcn(xFzg, xFzg_prev, yFzg, yFzg_prev)
% Prüfung ob Fzg eine Bewegung in X oder Y Richtung hat 
% X Bewegung: bewegung = 1
% Y Bewegung: bewegung = 2
% X&Y Bewegung: bewegung = 3
% Keine Bewegung: bewegung = 0

    if xFzg ~= xFzg_prev
        xBewegung = 1;
    else
        xBewegung = 0;
    end

    if yFzg  ~= yFzg_prev
        yBewegung = 2;
    else
        yBewegung = 0;
    end

    bewegung = xBewegung + yBewegung;

end

== matlab function FAS_Kreuzungswarner_Simulation_V1/Sensor B/Sensor Switch ==
  data: selection input; distance output; distanceK input; collisionK input; relevanzK input; distanceR input; collisionR input; relevanzR input; collision output; relevanz output
function [distance, collision, relevanz] = sensorSwitch(selection, ...
                                                        distanceK, collisionK, relevanzK, ...
                                                        distanceR, collisionR, relevanzR)
   

    switch selection

        case 1
            distance = distanceR;
            collision = collisionR;
            relevanz = relevanzR;

        case 2
            distance = distanceK;
            collision = collisionK;
            relevanz = relevanzK;

        % Wenn kein Sensor ausgewält ist
        case 3
            distance = 500;
            collision = 0;
            relevanz = 0;         
        
        % Fehler
        otherwise
            distance = -100;
            collision = -100;
            relevanz = -100;
    end
end

== matlab function FAS_Kreuzungswarner_Simulation_V1/Sensor Data Fusion /Verarbeitung Abstand ==
  data: distanceA input; distance output; distanceB input; defaultDistance parameter
function distance  = abstandsVerarbeitung(distanceA, distanceB, defaultDistance)
% Funktion zum Prüfen der Zwei Abstände A und B.
% A == B Output: A
% A <= B Output: A
% A >= B Output: B
% else   Output: defaultDistance

    if distanceA == distanceB
        distance = distanceA;
        return;
    elseif distanceA < distanceB
        distance = distanceA;
        return;
    elseif distanceA > distanceB
        distance = distanceB;
        return;
    else
        distance = defaultDistance;
    end
end

== matlab function FAS_Kreuzungswarner_Simulation_V1/Sensor Data Fusion /Verarbeitung Relevanz ==
  data: relevanzA input; relevanz output; relevanzB input
function relevanz  = abstandsVerarbeitung(relevanzA, relevanzB)
% Verarbeitung der zwei Relevanz Datan A und B
    
    % 0-Abfrage 
    % Wenn Sensor 0 ausgibt erkennt er kein Fzg
   
    if relevanzA == 0 && relevanzB == 0
        relevanz = 0;
        return;
    elseif relevanzA == 0 && relevanzB ~= 0
        relevanz = relevanzB;
        return;
    elseif relevanzA ~= 0 && relevanzB == 0
        relevanz = relevanzA;
        return;
    end

    % (1/-1)-Abfrage 
    % 1:    Relevantes Fzg
    % -1:   irelelvantes Fzg
    % 1 ist die dominate Relevanz
    
    if relevanzA == relevanzB
        relevanz = relevanzA;
        return;
    elseif relevanzA < relevanzB
        relevanz = relevanzB;
        return;
    elseif relevanzA > relevanzB
        relevanz = relevanzA;
        return;
    else
        relevanz = -100; % Error 
    end
end

== matlab function FAS_Kreuzungswarner_Simulation_V1/Sensor Data Fusion /Zusammenführung ==
  data: distanceI input; distanceO output; relevanz input; defaultDistance parameter
function distanceO = fcn(distanceI, relevanz, defaultDistance)
% Zusammenführen von Relevanz und Abstand
% Wenn eine Relevanz vorhanden (Relevanz = 1) ist soll der Abstand ausgegeben werden
    if relevanz == 1
        distanceO = distanceI;
    elseif relevanz == -1 || relevanz == 0
        distanceO = defaultDistance;
    else
        distanceO = defaultDistance; 
    end
end

== matlab function FAS_Kreuzungswarner_Simulation_V1/FAF/Berechnung Reaktion ==
  settings: updateMethod=DISCRETE
  data: GeschwindigkeitEGO input; Abstand input; Abstand_Memory input; Kollision input; Warnung output; Bremsverzoegerung output; Bremssignal output; PassiveSicherheit output; Airbag output; mutrocken parameter; munass parameter; g parameter; Haltezeit parameter; dt parameter; Ausloesezeit parameter; Airbagzeit parameter; Wetter input; muschnee parameter
%% Fahrerassistenzfunktion

% In dieser Funktion werden in Abhängigkeit aller Input-Parameter die
% entsprechenden Reaktionen berechnet. Es wird solange der Bremsweg
% berechnet bis das Auto anfängt zu Bremsen. In Abhängigkeit des Bremswegs
% und der verbleibenden Zeit werden dann entsprechend Reaktionen getroffen. 

function [Warnung, Bremsverzoegerung, Bremssignal, PassiveSicherheit, Airbag] = fcn(GeschwindigkeitEGO, Abstand, Abstand_Memory, Kollision, mutrocken, munass, g, Haltezeit, dt, Ausloesezeit, Airbagzeit, Wetter, muschnee)
    
    persistent Haltezeitcounter Bremsweg BremsflagStatus
    
    % Wetterbedingungen
    mu = mutrocken;
    if Wetter == 2
        mu = munass;
    elseif Wetter == 3
        mu = muschnee;
    end
    
    % Flags initialisieren
    Warnungflag = 0;
    Bremsflag = 0;
    PassiveSicherheitflag = 0;
    Airbagflag = 0;
           
    if isempty(Haltezeitcounter)
        Haltezeitcounter = 0;
    end
    
    % Bremsweg und maximale Verzögerung berechnen
    maxBremsBeschleunigung = mu * g;
    
    if isempty(Bremsweg)
        Bremsweg = 0;
        BremsflagStatus = 0; 
    end

    % Fallunterscheidung bei niedrigen Geschwindigkeiten (unter 30 km/h)
    if(GeschwindigkeitEGO < 8)    
        if BremsflagStatus == 0 && Abstand >= 4 * GeschwindigkeitEGO^2 / (2 * mu * g)
            Bremsweg = GeschwindigkeitEGO^2 / (2 * mu * g);
        else
            BremsflagStatus = 1;
        end
    else  
        if BremsflagStatus == 0 && Abstand >= 2 * GeschwindigkeitEGO^2 / (2 * mu * g)
            Bremsweg = GeschwindigkeitEGO^2 / (2 * mu * g);
        else
            BremsflagStatus = 1;
        end
    end
    
    %Flags berechnen:
    if (GeschwindigkeitEGO <= 8)
        if(Abstand - 6 * Bremsweg <= 0)
            Warnungflag = 1;
        end
    else
        if(Abstand - 3 * Bremsweg <= 0)
            Warnungflag = 1;
        end
    end
    
    if (GeschwindigkeitEGO <= 8)
        if(Abstand - 4 * Bremsweg <= 0) 
            Bremsflag = 1;
            if (GeschwindigkeitEGO == 0)
                Haltezeitcounter = Haltezeitcounter + 1;
            end
            if (Abstand > Abstand_Memory) && Haltezeitcounter > Haltezeit / dt
                Bremsflag = 0;
            end
        end
    else    
        if(Abstand - 2 * Bremsweg <= 0) 
            Bremsflag = 1;
            if (GeschwindigkeitEGO == 0)
                Haltezeitcounter = Haltezeitcounter + 1;
            end
            if (Abstand > Abstand_Memory) && Haltezeitcounter > Haltezeit / dt
                Bremsflag = 0;
            end
        end
    end
    
    if GeschwindigkeitEGO > 0.1 && Abstand / GeschwindigkeitEGO <= Ausloesezeit
        PassiveSicherheitflag = 1;
        if (Abstand / GeschwindigkeitEGO <= Airbagzeit)
            Airbagflag = 1;
        end
    elseif Abstand == 0
        PassiveSicherheitflag = 1;
        Airbagflag = 1;
    end
    
    % Auslösen des Airbags im Falle einer Kollision
    if (Kollision > 0)
        Airbagflag  = 1;
    end
        
    %Ausgabe
    Warnung = Warnungflag;
    Bremssignal = Bremsflag;
    PassiveSicherheit = PassiveSicherheitflag;
    Airbag = Airbagflag;
    Bremsverzoegerung = -maxBremsBeschleunigung;
end
